simulink model "car_sim"  (R2021b)
settings: Solver=FixedStepAuto  StartTime=0  StopTime=40  FixedStep=0.001  RelTol=1e-3
InitFcn:
  | init_car_dynamic
StopFcn:
  | plot_traj_results
values from neighbouring files (symbols this model uses):
  out = [ans.X.Data,ans.Y.Data,ans.psi_unwrap.Data,ans.omega.Data]    [init_car_dynamic.m]
  traj = [0 0 2.60589046157e-16 0.303981577543 1.60812264968e-16 -1 -1.60812264968e-16 1 0.0699968596385 0.000744733934178 0.0212771669454 0.303887540403 ... (7960 elements, 8x995)]    [traj_diy.mat]
  vx = 5    [init_car_dynamic.m]
undefined symbols (not defined in the file or in its folder): ctrl_K, ModelParams
libraries: slpidlib x3
settings Model: PacingRate=1000  Creator=Manny  LastModifiedBy=User
settings DataIOCC: SaveFormat=StructureWithTime
settings OptimizationCC: BlockReduction=off  BufferReuse=off
settings DebuggingCC: AlgebraicLoopMsg=none  UnconnectedInputMsg=none  UnconnectedOutputMsg=none  UnconnectedLineMsg=none  SFMachineParentedDataDiag=warning

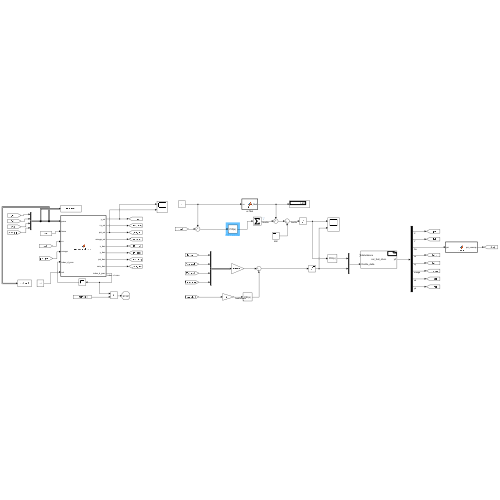
[thumbnail: Simulink's stored preview of the top-level diagram]
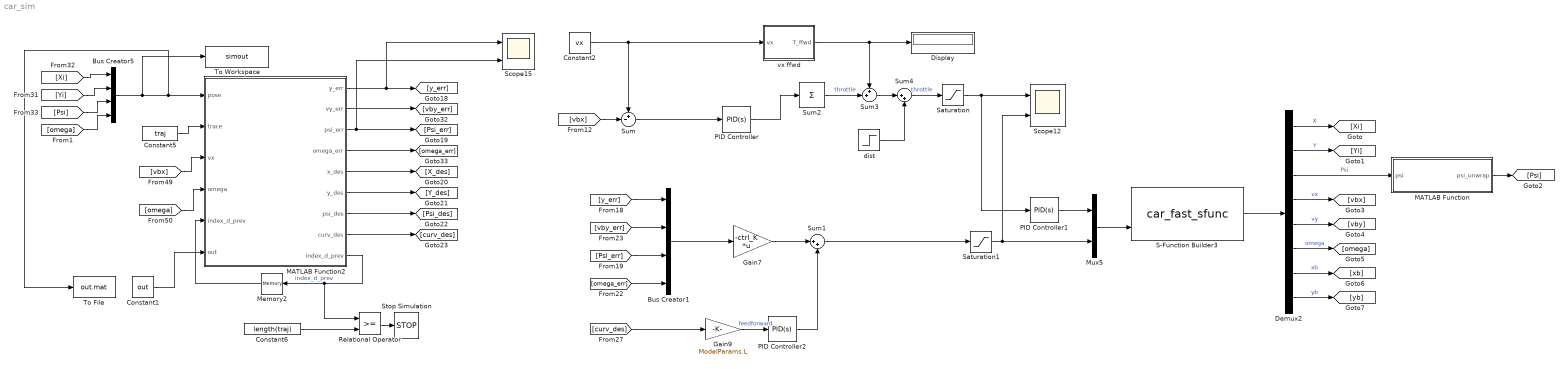
== system car_sim ==
  Bus Creator1 : BusCreator  Inputs=4
  Bus Creator5 : BusCreator  Inputs=4
  Constant1 : Constant  Value=out
  Constant2 : Constant  Value=vx
  Constant5 : Constant  Value=traj
  Constant6 : Constant  Value=length(traj)
  Demux2 : Demux  Outputs=8
  Display : Display
  Gain7 : Gain  Gain=-ctrl_K  Multiplication=Matrix(K*u) (u vector)
  Gain9 : Gain  Gain=ModelParams.L
  MATLAB Function : MATLAB Function  TreatAsAtomicUnit=on
  MATLAB Function2 : MATLAB Function  TreatAsAtomicUnit=on
  Memory2 : Memory
  Mux5 : Mux  Inputs=2
  PID Controller : slpidlib/PID Controller  Controller=PID  Form=Parallel  TimeDomain=Continuous-time  UseExternalTs=off  SampleTime=-1  IntegratorMethod=Forward Euler  FilterMethod=Forward Euler  ControllerParametersSource=internal  P=10  I=0  D=0  UseFilter=on  N=100  TunerSelectOption=Transfer Function Based (PID Tuner App)  InitialConditionSource=internal  InitialConditionForIntegrator=0  InitialConditionForFilter=0  DifferentiatorICPrevScaledInput=0  ExternalReset=none  TrackingMode=off  Kt=1  LimitOutput=off  SatLimitsSource=internal  UpperSaturationLimit=inf  LowerSaturationLimit=-inf  LinearizeAsGain=on  AntiWindupMode=none  Kb=1  POutMin=[]  POutMax=[]  IOutMin=[]  IOutMax=[]  DOutMin=[]  DOutMax=[]  NOutMin=[]  NOutMax=[]  SumOutMin=[]  SumOutMax=[]  SaturationOutMin=[]  SaturationOutMax=[]  PParamMin=[]  PParamMax=[]  IParamMin=[]  IParamMax=[]  DParamMin=[]  DParamMax=[]  NParamMin=[]  NParamMax=[]  KbParamMin=[]  KbParamMax=[]  KtParamMin=[]  KtParamMax=[]  KbOutMin=[]  KbOutMax=[]  KtOutMin=[]  KtOutMax=[]  IntegratorOutMin=[]  IntegratorOutMax=[]  FilterOutMin=[]  FilterOutMax=[]  SumI1OutMin=[]  SumI1OutMax=[]  SumI2OutMin=[]  SumI2OutMax=[]  SumI3OutMin=[]  SumI3OutMax=[]  SumI4OutMin=[]  SumI4OutMax=[]  SumDOutMin=[]  SumDOutMax=[]  DifferentiatorOutMin=[]  DifferentiatorOutMax=[]  FilterDiffOutCoefMin=[]  FilterDiffOutCoefMax=[]  ReciprocalOutMin=[]  ReciprocalOutMax=[]  SumDenOutMin=[]  SumDenOutMax=[]  SumNumOutMin=[]  SumNumOutMax=[]  DivideOutMin=[]  DivideOutMax=[]  UdiffTsProdOutMin=[]  UdiffTsProdOutMax=[]  NTsProdOutMin=[]  NTsProdOutMax=[]  UintegralTsProdOutMin=[]  UintegralTsProdOutMax=[]  UngainTsProdOutMin=[]  UngainTsProdOutMax=[]  IntegratorContinuousStateAttributes=''  IntegratorStateMustResolveToSignalObject=off  IntegratorRTWStateStorageClass=Auto  FilterContinuousStateAttributes=''  FilterStateMustResolveToSignalObject=off  FilterRTWStateStorageClass=Auto  ParallelPVariant=InternalParameters  IdealPVariant=Disabled  IVariant=InternalParameters  DVariant=InternalParameters  IntegratorVariant=Continuous  SatVariant=Disabled  AWVariant=Passthrough  PCopyVariant=Disabled  TRVariant=Disabled  FdbkBlocksVariant=Forward  IdealPFdbkVariant=Disabled  SatFdbkVariant=Disabled  DerivativeFilterVariant=ContFilter  NVariant=InternalParameters  NCopyVariant=Disabled  FilterICVariant=InternalICsFilter  IntegratorICVariant=InternalICs  ExternalResetVariant=Disabled  TRSumVariant=Passthrough  SumFdbkVariant=Disabled  SumVariant=Sum_PID  TsampFilterVariant=InternalTs  TsampNgainVariant=Passthrough  TsampIntegralVariant=Passthrough  ExternalSaturationOutDataTypeStr=Inherit: Same as second input
  PID Controller1 : slpidlib/PID Controller  Controller=PID  Form=Parallel  TimeDomain=Continuous-time  UseExternalTs=off  SampleTime=-1  IntegratorMethod=Forward Euler  FilterMethod=Forward Euler  ControllerParametersSource=internal  P=6  I=0.1  D=4  UseFilter=on  N=100  TunerSelectOption=Transfer Function Based (PID Tuner App)  InitialConditionSource=internal  InitialConditionForIntegrator=0  InitialConditionForFilter=0  DifferentiatorICPrevScaledInput=0  ExternalReset=none  TrackingMode=off  Kt=1  LimitOutput=off  SatLimitsSource=internal  UpperSaturationLimit=inf  LowerSaturationLimit=-inf  LinearizeAsGain=on  AntiWindupMode=none  Kb=1  POutMin=[]  POutMax=[]  IOutMin=[]  IOutMax=[]  DOutMin=[]  DOutMax=[]  NOutMin=[]  NOutMax=[]  SumOutMin=[]  SumOutMax=[]  SaturationOutMin=[]  SaturationOutMax=[]  PParamMin=[]  PParamMax=[]  IParamMin=[]  IParamMax=[]  DParamMin=[]  DParamMax=[]  NParamMin=[]  NParamMax=[]  KbParamMin=[]  KbParamMax=[]  KtParamMin=[]  KtParamMax=[]  KbOutMin=[]  KbOutMax=[]  KtOutMin=[]  KtOutMax=[]  IntegratorOutMin=[]  IntegratorOutMax=[]  FilterOutMin=[]  FilterOutMax=[]  SumI1OutMin=[]  SumI1OutMax=[]  SumI2OutMin=[]  SumI2OutMax=[]  SumI3OutMin=[]  SumI3OutMax=[]  SumI4OutMin=[]  SumI4OutMax=[]  SumDOutMin=[]  SumDOutMax=[]  DifferentiatorOutMin=[]  DifferentiatorOutMax=[]  FilterDiffOutCoefMin=[]  FilterDiffOutCoefMax=[]  ReciprocalOutMin=[]  ReciprocalOutMax=[]  SumDenOutMin=[]  SumDenOutMax=[]  SumNumOutMin=[]  SumNumOutMax=[]  DivideOutMin=[]  DivideOutMax=[]  UdiffTsProdOutMin=[]  UdiffTsProdOutMax=[]  NTsProdOutMin=[]  NTsProdOutMax=[]  UintegralTsProdOutMin=[]  UintegralTsProdOutMax=[]  UngainTsProdOutMin=[]  UngainTsProdOutMax=[]  IntegratorContinuousStateAttributes=''  IntegratorStateMustResolveToSignalObject=off  IntegratorRTWStateStorageClass=Auto  FilterContinuousStateAttributes=''  FilterStateMustResolveToSignalObject=off  FilterRTWStateStorageClass=Auto  ParallelPVariant=InternalParameters  IdealPVariant=Disabled  IVariant=InternalParameters  DVariant=InternalParameters  IntegratorVariant=Continuous  SatVariant=Disabled  AWVariant=Passthrough  PCopyVariant=Disabled  TRVariant=Disabled  FdbkBlocksVariant=Forward  IdealPFdbkVariant=Disabled  SatFdbkVariant=Disabled  DerivativeFilterVariant=ContFilter  NVariant=InternalParameters  NCopyVariant=Disabled  FilterICVariant=InternalICsFilter  IntegratorICVariant=InternalICs  ExternalResetVariant=Disabled  TRSumVariant=Passthrough  SumFdbkVariant=Disabled  SumVariant=Sum_PID  TsampFilterVariant=InternalTs  TsampNgainVariant=Passthrough  TsampIntegralVariant=Passthrough  ExternalSaturationOutDataTypeStr=Inherit: Same as second input
  PID Controller2 : slpidlib/PID Controller  Controller=PID  Form=Parallel  TimeDomain=Continuous-time  UseExternalTs=off  SampleTime=-1  IntegratorMethod=Forward Euler  FilterMethod=Forward Euler  ControllerParametersSource=internal  P=30  I=0.1  D=5  UseFilter=on  N=50  TunerSelectOption=Transfer Function Based (PID Tuner App)  InitialConditionSource=internal  InitialConditionForIntegrator=0  InitialConditionForFilter=0  DifferentiatorICPrevScaledInput=0  ExternalReset=none  TrackingMode=off  Kt=1  LimitOutput=off  SatLimitsSource=internal  UpperSaturationLimit=inf  LowerSaturationLimit=-inf  LinearizeAsGain=on  AntiWindupMode=none  Kb=1  POutMin=[]  POutMax=[]  IOutMin=[]  IOutMax=[]  DOutMin=[]  DOutMax=[]  NOutMin=[]  NOutMax=[]  SumOutMin=[]  SumOutMax=[]  SaturationOutMin=[]  SaturationOutMax=[]  PParamMin=[]  PParamMax=[]  IParamMin=[]  IParamMax=[]  DParamMin=[]  DParamMax=[]  NParamMin=[]  NParamMax=[]  KbParamMin=[]  KbParamMax=[]  KtParamMin=[]  KtParamMax=[]  KbOutMin=[]  KbOutMax=[]  KtOutMin=[]  KtOutMax=[]  IntegratorOutMin=[]  IntegratorOutMax=[]  FilterOutMin=[]  FilterOutMax=[]  SumI1OutMin=[]  SumI1OutMax=[]  SumI2OutMin=[]  SumI2OutMax=[]  SumI3OutMin=[]  SumI3OutMax=[]  SumI4OutMin=[]  SumI4OutMax=[]  SumDOutMin=[]  SumDOutMax=[]  DifferentiatorOutMin=[]  DifferentiatorOutMax=[]  FilterDiffOutCoefMin=[]  FilterDiffOutCoefMax=[]  ReciprocalOutMin=[]  ReciprocalOutMax=[]  SumDenOutMin=[]  SumDenOutMax=[]  SumNumOutMin=[]  SumNumOutMax=[]  DivideOutMin=[]  DivideOutMax=[]  UdiffTsProdOutMin=[]  UdiffTsProdOutMax=[]  NTsProdOutMin=[]  NTsProdOutMax=[]  UintegralTsProdOutMin=[]  UintegralTsProdOutMax=[]  UngainTsProdOutMin=[]  UngainTsProdOutMax=[]  IntegratorContinuousStateAttributes=''  IntegratorStateMustResolveToSignalObject=off  IntegratorRTWStateStorageClass=Auto  FilterContinuousStateAttributes=''  FilterStateMustResolveToSignalObject=off  FilterRTWStateStorageClass=Auto  ParallelPVariant=InternalParameters  IdealPVariant=Disabled  IVariant=InternalParameters  DVariant=InternalParameters  IntegratorVariant=Continuous  SatVariant=Disabled  AWVariant=Passthrough  PCopyVariant=Disabled  TRVariant=Disabled  FdbkBlocksVariant=Forward  IdealPFdbkVariant=Disabled  SatFdbkVariant=Disabled  DerivativeFilterVariant=ContFilter  NVariant=InternalParameters  NCopyVariant=Disabled  FilterICVariant=InternalICsFilter  IntegratorICVariant=InternalICs  ExternalResetVariant=Disabled  TRSumVariant=Passthrough  SumFdbkVariant=Disabled  SumVariant=Sum_PID  TsampFilterVariant=InternalTs  TsampNgainVariant=Passthrough  TsampIntegralVariant=Passthrough  ExternalSaturationOutDataTypeStr=Inherit: Same as second input
  Relational Operator : RelationalOperator  OutDataTypeStr=boolean  RndMeth=Simplest
  S-Function Builder3 : S-Function  FunctionName=car_fast_sfunc  SFunctionModules=car_fast_sfunc_wrapper  SFunctionDeploymentMode=off  EnableBusSupport=off  mask(S-Function Builder){}
      mask help: Simulink:masks:SFunctionBuilder_MD
      mask init:
      | val = [[.9  0.75 0.75 1 1 .9 .9 1]',[1 1 0.75 0.75 .9 .9 1 .9]'];try , sys = get_param(gcb,'SfunBuilderFcnName');if isempty(sys), sys = get_param(gcb,'FunctionName'); end,catch, sys = get_param(gcb,'FunctionName'); end
      settings: CopyFcn=set_param(gcbh,'LinkStatus','none')  OpenFcn=sfunctionwizard(gcbh)
      mask Display: plot(val(:,1),val(:,2)),disp(sys),port_label('input',1,'disturbance'),port_label('input',2,'throttle_delta'),port_label('output',1,'y0')
  Saturation : Saturate  UpperLimit=1  LowerLimit=0
  Saturation1 : Saturate  UpperLimit=pi/3  LowerLimit=-pi/3
  Scope12 : Scope  NumInputPorts=2
  Scope15 : Scope  NumInputPorts=2
  Stop Simulation : Stop
  Sum : Sum  Inputs=+-|
  Sum1 : Sum  Inputs=|++
  Sum2 : Sum  Inputs=+
  Sum3 : Sum  Inputs=++|
  Sum4 : Sum  Inputs=|++
  To File : ToFile  Filename=out.mat  SaveFormat=Timeseries
  To Workspace : ToWorkspace  VariableName=simout  SaveFormat=Timeseries  SampleTime=-1
  dist : Step  After=-0.05  SampleTime=0
  vx ffwd : MATLAB Function  TreatAsAtomicUnit=on
  wires:
  S-Function Builder3/1 -> Demux2/1
  Mux5/1 -> S-Function Builder3/2
  Gain7/1 -> Sum1/1
  Demux2/1 -> [Xi]  "X"
  Demux2/2 -> [Yi]  "Y"
  Demux2/3 -> MATLAB Function/1(psi)  "Psi"
  Demux2/4 -> [vbx]  "vx"
  Demux2/5 -> [vby]  "vy"
  Demux2/6 -> [omega]  "omega"
  Demux2/7 -> [xb]  "xb"
  Demux2/8 -> [yb]  "yb"
  [vby_err] -> Bus Creator1/2
  [omega_err] -> Bus Creator1/4
  Bus Creator1/1 -> Gain7/1
  [vbx] -> Sum/2
  [y_err] -> Bus Creator1/1
  [Psi_err] -> Bus Creator1/3
  [curv_des] -> Gain9/1
  MATLAB Function/1(psi_unwrap) -> [Psi]
  [Yi] -> Bus Creator5/2
  [Xi] -> Bus Creator5/1
  Bus Creator5/1 -> To Workspace/1, To File/1, MATLAB Function2/1(pose)
  Constant5/1 -> MATLAB Function2/2(trace)
  [Psi] -> Bus Creator5/3
  MATLAB Function2/5(x_des) -> [X_des]
  MATLAB Function2/7(psi_des) -> [Psi_des]
  MATLAB Function2/6(y_des) -> [Y_des]
  MATLAB Function2/8(curv_des) -> [curv_des]
  MATLAB Function2/9(index_d_prev) -> Relational Operator/1, Memory2/1  "index_d_prev"
  Memory2/1 -> MATLAB Function2/5("index_d_prev ")
  MATLAB Function2/1(y_err) -> [y_err], Scope15/1
  MATLAB Function2/3(psi_err) -> [Psi_err], Scope15/2
  Relational Operator/1 -> Stop Simulation/1
  Constant6/1 -> Relational Operator/2
  vx ffwd/1(T_ffwd) -> Sum3/1, Display/1
  Sum2/1 -> Sum3/2  "throttle"
  Sum3/1 -> Sum4/1
  Sum4/1 -> Saturation/1  "throttle"
  dist/1 -> Sum4/2
  [vbx] -> MATLAB Function2/3(vx)
  [omega] -> MATLAB Function2/4(omega)
  MATLAB Function2/4(omega_err) -> [omega_err]
  MATLAB Function2/2(vy_err) -> [vby_err]
  PID Controller/1 -> Sum2/1
  Sum/1 -> PID Controller/1
  Constant2/1 -> vx ffwd/1(vx), Sum/1
  Saturation1/1 -> Mux5/2, Scope12/2
  Sum1/1 -> Saturation1/1
  Gain9/1 -> PID Controller2/1  "feedforward"
  PID Controller2/1 -> Sum1/2
  Constant1/1 -> MATLAB Function2/6(out)
  [omega] -> Bus Creator5/4
  Saturation/1 -> PID Controller1/1, Scope12/1
  PID Controller1/1 -> Mux5/1

== matlab function car_sim/MATLAB Function ==
  data: psi input; psi_unwrap output
function psi_unwrap = unwrap(psi)

if ( psi > pi)
    psi = psi - 2*pi;
end

if( psi <= -pi)
    psi = psi + 2*pi;
end

psi_unwrap = psi;

== matlab function car_sim/MATLAB Function2 ==
  data: y_err output; vy_err output; psi_err output; omega_err output; pose input; trace input; vx input; omega input; x_des output; y_des output; psi_des output; curv_des output; index_d_prev input; index_d_prev output; out input
function [y_err,vy_err,psi_err,omega_err,x_des,y_des,psi_des,curv_des, index_d_prev]=cal_nearest_index(pose, trace, vx, omega, index_d_prev,out)

traj_x=trace(1,:);      %给定x坐标
traj_y=trace(2,:);      %给定y坐标
traj_psi=trace(3,:);    %给定航向角Psi
traj_k=trace(4,:);      %曲率
% traj_x=out(:,1)';      %给定x坐标
% traj_y=out(:,2)';      %给定y坐标
% traj_psi=out(:,3)';    %给定航向角Psi
% traj_k=out(:,4)';      %曲率

x = pose(1);
y = pose(2);
psi = pose(3);

dx=x*ones(1,length(traj_x))-traj_x;
dy=y*ones(1,length(traj_y))-traj_y;

% find the nearest index
d=dx.^2+dy.^2;
[mini_d,index_d]=min(d);

% go forward
if index_d <= index_d_prev
    index_d = index_d_prev;
end

index_d_prev = index_d;
dis=sqrt(mini_d);

% current position point to designed positon
dx1=traj_x(index_d)-x;
dy1=traj_y(index_d)-y;

% yaw vector [cos(psi_des) sin(psi_des)]
axis = cross([dx1 dy1 1], [cos(traj_psi(index_d)) sin(traj_psi(index_d)) 1]);

if axis(3)<0
    dis=-dis;
end

psi_des = pi_2_pi(traj_psi(index_d));
x_des = traj_x(index_d);
y_des = traj_y(index_d);
curv_des = traj_k(index_d);

psi_err = psi - psi_des;
psi_err = pi_2_pi(psi_err);
y_err = dis;

% give a better vy_err and omega_err
% vy_err = vx*cos(psi_err);
% omega_des = vx*curv_des;
% omega_err = omega - omega_des;

vy_err = 2*y_err;
omega_err = 2*psi_err;

end

function angle=pi_2_pi(angle)
if angle > pi
    angle=angle-2*pi;
elseif angle < -pi
    angle=angle+2*pi;
end
end

== matlab function car_sim/vx ffwd ==
  data: vx input; T_ffwd output
function T_ffwd = fcn(vx)

m = 0.041;
g = 9.8;
Iz = 27.8e-6;
lf = 0.029;
lr = 0.033;
Cm1=0.287;
Cm2=0.0545;
Cr0=0.0218;
Cr2=0.00035;

Nf = m*g*lr/(lf+lr);
Nr = m*g*lf/(lf+lr);

T_ffwd = -(-Cr0*m*g-2*Cr2*vx^2)/(Cm1-Cm2*vx);
